simulink model "torqueBalancingJointControl"  (Simulink 8.0)
settings: Solver=FixedStepDiscrete  StartTime=0.0  StopTime=simulationTime  FixedStep=Ts  RelTol=1e-3
InitFcn:
  | initTorqueBalancingJc;
values from neighbouring files (symbols this model uses):
  WBT_modelName = 'matlabTorqueBalancing'    [initTorqueBalancing.m]
undefined symbols (not defined in the file or in its folder): bVectorConstraints, ConstraintsMatrix, DiscIntNeverNeededParam, gain, LEFT_RIGHT_FOOT_IN_CONTACT, reg, ROBOT_DOF, ROBOT_DOF_FOR_SIMULINK, sat, Ts
libraries: WBToolboxLibrary x56, simulink x2
settings Model: Creator=daniele  LastModifiedBy=gnava
settings DebuggingCC: FcnCallInpInsideContextMsg=EnableAllAsWarning  FrameProcessingCompatibilityMsg=error
settings SFSimCC: SimParseCustomCode=off
settings CodeAppCC: CustomSymbolStrType=$N$R$M_T
settings GRTTargetCC: CodeReplacementLibrary=C89/C90 (ANSI)  CombineOutputUpdateFcns=off  GRTInterface=on

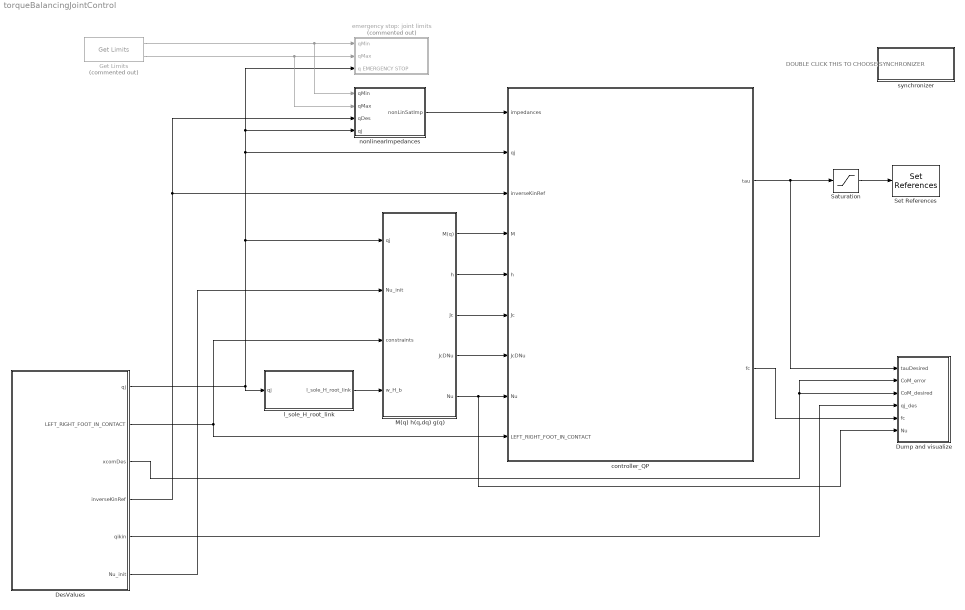
== system torqueBalancingJointControl ==
  note: DOUBLE CLICK THIS TO
      |  CHOOSE SYNCHRONIZER
  DesValues : Subsystem
  Dump and visualize : Subsystem
  Get Limits : WBToolboxLibrary/wholeBodyStates/Get Limits  Commented=on  limitsType=Position  robotName=WBT_robotName  localName=WBT_modelName  wbiFile=WBT_wbiFilename  wbiList=WBT_wbiList
  M(q) h(q,dq) g(q) : Subsystem
  Saturation : Saturate  UpperLimit=sat.torque  LowerLimit=-sat.torque
  Set References : WBToolboxLibrary/wholeBodyActuators/Set References  controlType=Torque  robotName=WBT_robotName  localName=WBT_modelName  wbiFile=WBT_wbiFilename  wbiList=WBT_wbiList
  controller_QP : Subsystem
  emergency stop: joint limits : Subsystem  Commented=on
  l_sole_H_root_link : Subsystem
  nonlinearImpedances : Subsystem
  synchronizer : Subsystem
  wires:
  DesValues/1(qj) -> l_sole_H_root_link/1(qj), M(q) h(q,dq) g(q)/1(qj), controller_QP/2(qj), nonlinearImpedances/4(qj), emergency stop: joint limits/3(q EMERGENCY STOP)
  M(q) h(q,dq) g(q)/1(M(q)) -> controller_QP/4(M)
  Get Limits/1 -> nonlinearImpedances/1(qMin), emergency stop: joint limits/1(qMin)
  M(q) h(q,dq) g(q)/2(h) -> controller_QP/5(h)
  controller_QP/1("tau ") -> Saturation/1, Dump and visualize/1(tauDesired)
  Saturation/1 -> Set References/1
  DesValues/2(LEFT_RIGHT_FOOT_IN_CONTACT) -> controller_QP/9(LEFT_RIGHT_FOOT_IN_CONTACT), M(q) h(q,dq) g(q)/3(constraints)
  nonlinearImpedances/1(nonLinSatImp) -> controller_QP/1(impedances)
  M(q) h(q,dq) g(q)/5(Nu) -> Dump and visualize/6(Nu), controller_QP/8(Nu)
  M(q) h(q,dq) g(q)/3(Jc) -> controller_QP/6(Jc)
  M(q) h(q,dq) g(q)/4(JcDNu) -> controller_QP/7(JcDNu)
  DesValues/4(inverseKinRef) -> controller_QP/3(inverseKinRef), nonlinearImpedances/3(qDes)
  DesValues/5(qikin) -> Dump and visualize/4(qj_des)
  DesValues/3(xcomDes) -> Dump and visualize/2(CoM_error), Dump and visualize/3(CoM_desired)
  controller_QP/2(fc) -> Dump and visualize/5(fc)
  Get Limits/2 -> nonlinearImpedances/2(qMax), emergency stop: joint limits/2(qMax)
  l_sole_H_root_link/1(l_sole_H_root_link) -> M(q) h(q,dq) g(q)/4(w_H_b)
  DesValues/6(Nu_init) -> M(q) h(q,dq) g(q)/2(Nu_init)

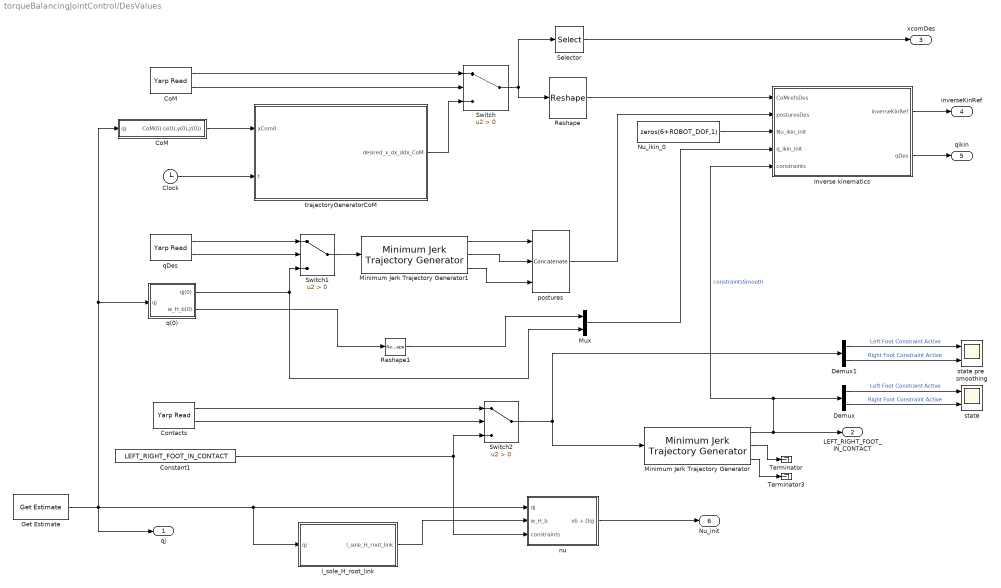
== system torqueBalancingJointControl/DesValues ==
  Clock : Clock
  CoM : WBToolboxLibrary/Utilities/Yarp Read  portName=['/' WBT_modelName '/comDes:i']  signalSize=9  blocking=off  timestamp=off  autoconnect=off  errorOnConnection=on
  "CoM " : Subsystem
  Constant1 : Constant  Value=LEFT_RIGHT_FOOT_IN_CONTACT
  Contacts : WBToolboxLibrary/Utilities/Yarp Read  portName=['/' WBT_modelName '/constraints:i']  signalSize=2  blocking=off  timestamp=off  autoconnect=off  errorOnConnection=on
  Demux : Demux  Outputs=2
  Demux1 : Demux  Outputs=2
  Get Estimate : WBToolboxLibrary/wholeBodyStates/Get Estimate  estimateType=Joints Position  robotName=WBT_robotName  localName=WBT_modelName  wbiFile=WBT_wbiFilename  wbiList=WBT_wbiList
  Inverse kinematics : Subsystem
  Minimum Jerk Trajectory Generator : WBToolboxLibrary/Utilities/Minimum Jerk Trajectory Generator  externalSettlingTime=off  settlingTime=3  sampleTime=Ts  firstDerivatives=on  secondDerivatives=on  explicitInitialValue=off
  Minimum Jerk Trajectory Generator1 : WBToolboxLibrary/Utilities/Minimum Jerk Trajectory Generator  externalSettlingTime=off  settlingTime=3  sampleTime=Ts  firstDerivatives=on  secondDerivatives=on  explicitInitialValue=off
  Mux : Mux  Inputs=2
  Nu_ikin_0 : Constant  Value=zeros(6+ROBOT_DOF,1)
  Reshape : Reshape  OutputDimensionality=Customize  OutputDimensions=[3,3]
  Reshape1 : Reshape
  Selector : Selector  InputPortWidth=9  IndexOptions=Index vector (dialog)  Indices=[1:3]  OutputSizes=1
  Switch : Switch  Criteria=u2 > Threshold
  Switch1 : Switch  Criteria=u2 > Threshold
  Switch2 : Switch  Criteria=u2 > Threshold
  Terminator : Terminator
  Terminator3 : Terminator
  l_sole_H_root_link : Subsystem
  nu : Subsystem
  postures : Concatenate  NumInputs=3  Mode=Multidimensional array  ConcatenateDimension=2
  q(0) : Subsystem
  qDes : WBToolboxLibrary/Utilities/Yarp Read  portName=['/' WBT_modelName '/qDes:i']  signalSize=ROBOT_DOF  blocking=off  timestamp=off  autoconnect=off  errorOnConnection=on
  state : Scope  NumInputPorts=2
      settings: ShowLegends=on  TimeRange=60  YMin=0~0  YMax=2~2
  state pre  smoothing : Scope  NumInputPorts=2
      settings: ShowLegends=on  TimeRange=60  YMin=0~0  YMax=2~2  SaveName=ScopeData7
  trajectoryGeneratorCoM : MATLAB Function  TreatAsAtomicUnit=on
  qj : Outport
  LEFT_RIGHT_FOOT_IN_CONTACT : Outport  Port=2
  xcomDes : Outport  Port=3
  inverseKinRef : Outport  Port=4
  qikin : Outport  Port=5
  Nu_init : Outport  Port=6
  wires:
  Constant1/1 -> Switch2/3, nu/3("constraints ")
  Minimum Jerk Trajectory Generator/1 -> Inverse kinematics/5(constraints), Demux/1, LEFT_RIGHT_FOOT_IN_CONTACT/1  "constraintsSmooth"
  CoM/2 -> Switch/2
  CoM/1 -> Switch/1
  Reshape/1 -> Inverse kinematics/1(CoMrefsDes)
  Switch/1 -> Reshape/1, Selector/1
  qDes/2 -> Switch1/2
  qDes/1 -> Switch1/1
  Selector/1 -> xcomDes/1
  Contacts/2 -> Switch2/2
  Contacts/1 -> Switch2/1
  Switch2/1 -> Demux1/1, Minimum Jerk Trajectory Generator/1
  Demux/1 -> state/1  "Left Foot Constraint Active"
  Demux/2 -> state/2  "Right Foot Constraint Active"
  Demux1/1 -> state pre  smoothing/1  "Left Foot Constraint Active"
  Demux1/2 -> state pre  smoothing/2  "Right Foot Constraint Active"
  "CoM "/1(CoM(0) (x(0),y(0),z(0))) -> trajectoryGeneratorCoM/1(xCom0)
  Clock/1 -> trajectoryGeneratorCoM/2(t)
  trajectoryGeneratorCoM/1(desired_x_dx_ddx_CoM) -> Switch/3
  Switch1/1 -> Minimum Jerk Trajectory Generator1/1
  Minimum Jerk Trajectory Generator1/1 -> postures/1
  Minimum Jerk Trajectory Generator1/2 -> postures/2
  Minimum Jerk Trajectory Generator1/3 -> postures/3
  Nu_ikin_0/1 -> Inverse kinematics/3(Nu_ikin_init)
  Mux/1 -> Inverse kinematics/4(q_ikin_init)
  q(0)/1(qj(0)) -> Mux/2, Switch1/3
  postures/1 -> Inverse kinematics/2(posturesDes)
  Inverse kinematics/2(qDes) -> qikin/1
  Minimum Jerk Trajectory Generator/2 -> Terminator/1
  Minimum Jerk Trajectory Generator/3 -> Terminator3/1
  q(0)/2(w_H_b(0)) -> Reshape1/1
  Reshape1/1 -> Mux/1
  nu/1(vb + Dqj) -> Nu_init/1
  l_sole_H_root_link/1(l_sole_H_root_link) -> nu/2(w_H_b)
  Get Estimate/1 -> qj/1, q(0)/1(qj), "CoM "/1(qj), l_sole_H_root_link/1(qj), nu/1(qj)
  Inverse kinematics/1(inverseKinRef) -> inverseKinRef/1

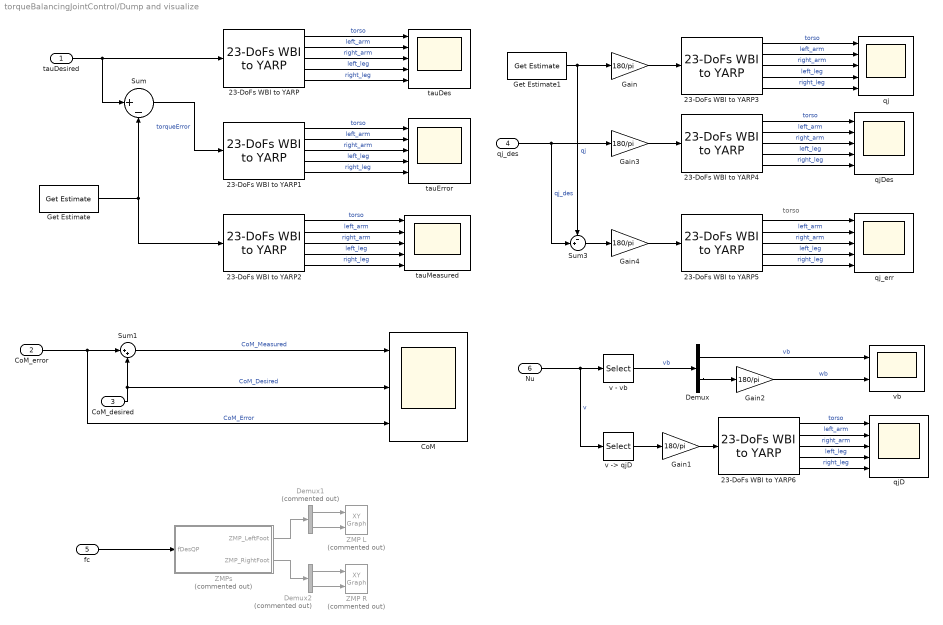
== system torqueBalancingJointControl/Dump and visualize ==
  note: torso
  tauDesired : Inport
  CoM_error : Inport  Port=2
  CoM_desired : Inport  Port=3
  qj_des : Inport  Port=4
  fc : Inport  Port=5
  Nu : Inport  Port=6
  23-DoFs WBI to YARP{,1..6} (7 alike) : WBToolboxLibrary/Utilities/23-DoFs WBI to YARP
  CoM : Scope  NumInputPorts=3
      settings: ShowLegends=on  TimeRange=400  YMin=-0.25~-0.2~-0.2  YMax=1.25~0.6~0.6  SaveName=CoM_data
  Demux : Demux  Outputs=2
  Demux1 : Demux  Commented=on  Outputs=2
  Demux2 : Demux  Commented=on  Outputs=2
  Gain{,1..4} (5 alike) : Gain  Gain=180/pi
  Get Estimate : WBToolboxLibrary/wholeBodyStates/Get Estimate  estimateType=Joints Torque  robotName=WBT_robotName  localName=WBT_modelName  wbiFile=WBT_wbiFilename  wbiList=WBT_wbiList
  Get Estimate1 : WBToolboxLibrary/wholeBodyStates/Get Estimate  estimateType=Joints Position  robotName=WBT_robotName  localName=WBT_modelName  wbiFile=WBT_wbiFilename  wbiList=WBT_wbiList
  Sum : Sum  Inputs=|+-
  Sum1 : Sum  Inputs=|++
  Sum3 : Sum  Inputs=-+|
  ZMP L : simulink/Sinks/XY Graph  Commented=on  xmin=gain.footSize(1,1)  xmax=gain.footSize(1,2)  ymin=gain.footSize(2,1)  ymax=gain.footSize(2,2)  st=-1
  ZMP R : simulink/Sinks/XY Graph  Commented=on  xmin=gain.footSize(1,1)  xmax=gain.footSize(1,2)  ymin=gain.footSize(2,1)  ymax=gain.footSize(2,2)  st=-1
  ZMPs : Subsystem  Commented=on
  qj : Scope  NumInputPorts=5
      settings: ShowLegends=on  TimeRange=40  YMin=-5~-40~-40~-15~-15  YMax=8~60~60~15~15  SaveName=qj_and_v
  qjD : Scope  NumInputPorts=5
      settings: ShowLegends=on  TimeRange=40  YMin=-1~-0.2~-0.6~-3~-3  YMax=3~0.5~0.3~3~3  SaveName=qj_and_v1
  qjDes : Scope  NumInputPorts=5
      settings: ShowLegends=on  TimeRange=40  YMin=-13.18879~-50.35129~-51.01363~-14.07847~-15.42592  YMax=8.56867~62.73253~62.72359~15.05436~15.88206  SaveName=qj_and_v3
  qj_err : Scope  NumInputPorts=5
      settings: ShowLegends=on  TimeRange=40  YMin=-27.27476~-4.23851~-4.57478~-6.37088~-5.38345  YMax=17.10367~4.06727~2.87419~5.35549~6.40509  SaveName=qj_and_v4
  tauDes : Scope  NumInputPorts=5
      settings: ShowLegends=on  TimeRange=14  YMin=-19.49982~-5.04916~-6.41013~-19.61704~-14.11485  YMax=15.70467~4.10511~5.2534~18.2484~18.38621  SaveName=tauDes
  tauError : Scope  NumInputPorts=5
      settings: ShowLegends=on  TimeRange=90  YMin=-4.41555~-1.22651~-0.86191~-3.55477~-4.30808  YMax=5.88399~0.83922~1.20608~5.47683~6.35708  SaveName=tauError
  tauMeasured : Scope  NumInputPorts=5
      settings: ShowLegends=on  TimeRange=14  YMin=-6~-2.5~-2.5~-6~-6  YMax=5~2~1.5~5~5  SaveName=tauMeasured
  v - vb : Selector  InputPortWidth=ROBOT_DOF+6  IndexOptions=Index vector (dialog)  Indices=[1:6]  OutputSizes=1
  "v -> qjD" : Selector  InputPortWidth=ROBOT_DOF+6  IndexOptions=Index vector (dialog)  Indices=[7:ROBOT_DOF+6]  OutputSizes=1
  vb : Scope  NumInputPorts=2
      settings: ShowLegends=on  TimeRange=40  YMin=-0.02~-1.75  YMax=0.0175~2  SaveName=qj_and_v2
  wires:
  CoM_error/1 -> CoM/3, Sum1/1  "CoM_Error"
  CoM_desired/1 -> Sum1/2, CoM/2  "CoM_Desired"
  Sum1/1 -> CoM/1  "CoM_Measured"
  Nu/1 -> "v -> qjD"/1, v - vb/1  "v"
  Get Estimate1/1 -> Sum3/1, Gain/1  "qj"
  Gain/1 -> 23-DoFs WBI to YARP3/1
  23-DoFs WBI to YARP3/5 -> qj/5  "right_leg"
  23-DoFs WBI to YARP3/1 -> qj/1  "torso"
  23-DoFs WBI to YARP3/2 -> qj/2  "left_arm"
  23-DoFs WBI to YARP3/4 -> qj/4  "left_leg"
  23-DoFs WBI to YARP3/3 -> qj/3  "right_arm"
  23-DoFs WBI to YARP6/5 -> qjD/5  "right_leg"
  23-DoFs WBI to YARP6/1 -> qjD/1  "torso"
  23-DoFs WBI to YARP6/2 -> qjD/2  "left_arm"
  23-DoFs WBI to YARP6/4 -> qjD/4  "left_leg"
  23-DoFs WBI to YARP6/3 -> qjD/3  "right_arm"
  "v -> qjD"/1 -> Gain1/1
  v - vb/1 -> Demux/1  "vb"
  Demux/1 -> vb/1  "vb"
  Demux/2 -> Gain2/1
  Gain1/1 -> 23-DoFs WBI to YARP6/1
  Gain2/1 -> vb/2  "wb"
  fc/1 -> ZMPs/1(fDesQP)
  ZMPs/1(ZMP_LeftFoot) -> Demux1/1
  ZMPs/2(ZMP_RightFoot) -> Demux2/1
  Demux1/1 -> ZMP L/1
  Demux1/2 -> ZMP L/2
  Demux2/1 -> ZMP R/1
  Demux2/2 -> ZMP R/2
  tauDesired/1 -> Sum/1, 23-DoFs WBI to YARP/1
  Get Estimate/1 -> 23-DoFs WBI to YARP2/1, Sum/2
  23-DoFs WBI to YARP/5 -> tauDes/5  "right_leg"
  23-DoFs WBI to YARP/1 -> tauDes/1  "torso"
  23-DoFs WBI to YARP/2 -> tauDes/2  "left_arm"
  23-DoFs WBI to YARP/4 -> tauDes/4  "left_leg"
  23-DoFs WBI to YARP/3 -> tauDes/3  "right_arm"
  23-DoFs WBI to YARP1/5 -> tauError/5  "right_leg"
  23-DoFs WBI to YARP1/1 -> tauError/1  "torso"
  23-DoFs WBI to YARP1/2 -> tauError/2  "left_arm"
  23-DoFs WBI to YARP1/4 -> tauError/4  "left_leg"
  23-DoFs WBI to YARP1/3 -> tauError/3  "right_arm"
  Sum/1 -> 23-DoFs WBI to YARP1/1  "torqueError"
  23-DoFs WBI to YARP2/5 -> tauMeasured/5  "right_leg"
  23-DoFs WBI to YARP2/1 -> tauMeasured/1  "torso"
  23-DoFs WBI to YARP2/2 -> tauMeasured/2  "left_arm"
  23-DoFs WBI to YARP2/4 -> tauMeasured/4  "left_leg"
  23-DoFs WBI to YARP2/3 -> tauMeasured/3  "right_arm"
  23-DoFs WBI to YARP4/5 -> qjDes/5  "right_leg"
  23-DoFs WBI to YARP4/1 -> qjDes/1  "torso"
  23-DoFs WBI to YARP4/2 -> qjDes/2  "left_arm"
  23-DoFs WBI to YARP4/4 -> qjDes/4  "left_leg"
  23-DoFs WBI to YARP4/3 -> qjDes/3  "right_arm"
  Gain4/1 -> 23-DoFs WBI to YARP5/1
  23-DoFs WBI to YARP5/5 -> qj_err/5  "right_leg"
  23-DoFs WBI to YARP5/2 -> qj_err/2  "left_arm"
  23-DoFs WBI to YARP5/4 -> qj_err/4  "left_leg"
  23-DoFs WBI to YARP5/3 -> qj_err/3  "right_arm"
  Sum3/1 -> Gain4/1
  qj_des/1 -> Gain3/1, Sum3/2  "qj_des"
  Gain3/1 -> 23-DoFs WBI to YARP4/1
  23-DoFs WBI to YARP5/1 -> qj_err/1

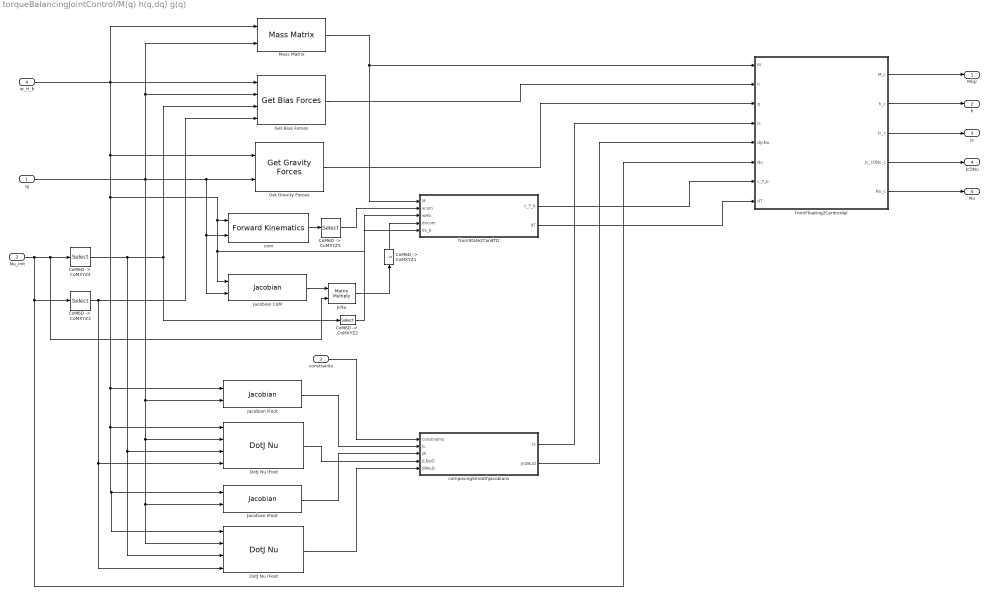
== system torqueBalancingJointControl/M(q) h(q,dq) g(q) ==
  qj : Inport
  Nu_init : Inport  Port=2
  constraints : Inport  Port=3
  w_H_b : Inport  Port=4
  "CoM6D ->  CoMXYZ1" : Selector  InputPortWidth=6  IndexOptions=Index vector (dialog)  Indices=[1 2 3]  OutputSizes=1
  "CoM6D ->  CoMXYZ2" : Selector  InputPortWidth=6  IndexOptions=Index vector (dialog)  Indices=[1 2 3]  OutputSizes=1
  "CoM6D ->  CoMXYZ3" : Selector  InputPortWidth=6+ROBOT_DOF  IndexOptions=Index vector (dialog)  Indices=[7:6+ROBOT_DOF]  OutputSizes=1
  "CoM6D ->  CoMXYZ4" : Selector  InputPortWidth=6+ROBOT_DOF  IndexOptions=Index vector (dialog)  Indices=[1 2 3 4 5 6]  OutputSizes=1
  "CoM6D ->  CoMXYZ5" : Selector  NumberOfDimensions=2  InputPortWidth=7  IndexOptions=Index vector (dialog),Index vector (dialog)  Indices=[1 2 3],[4]  OutputSizes=1,1
  DotJ Nu lFoot : WBToolboxLibrary/wholeBodyModel/Jacobians/DotJ Nu  frameName='l_sole'  robotName=WBT_robotName  localName=WBT_modelName  wbiFile=WBT_wbiFilename  wbiList=WBT_wbiList
  DotJ Nu rFoot : WBToolboxLibrary/wholeBodyModel/Jacobians/DotJ Nu  frameName='r_sole'  robotName=WBT_robotName  localName=WBT_modelName  wbiFile=WBT_wbiFilename  wbiList=WBT_wbiList
  Get Bias Forces : WBToolboxLibrary/wholeBodyModel/Dynamics/Get Bias Forces  robotName=WBT_robotName  localName=WBT_modelName  wbiFile=WBT_wbiFilename  wbiList=WBT_wbiList
  Get Gravity Forces : WBToolboxLibrary/wholeBodyModel/Dynamics/Get Gravity Forces  robotName=WBT_robotName  localName=WBT_modelName  wbiFile=WBT_wbiFilename  wbiList=WBT_wbiList
  Jacobian CoM : WBToolboxLibrary/wholeBodyModel/Jacobians/Jacobian  frameName='com'  robotName=WBT_robotName  localName=WBT_modelName  wbiFile=WBT_wbiFilename  wbiList=WBT_wbiList
  Jacobian lFoot : WBToolboxLibrary/wholeBodyModel/Jacobians/Jacobian  frameName='l_sole'  robotName=WBT_robotName  localName=WBT_modelName  wbiFile=WBT_wbiFilename  wbiList=WBT_wbiList
  Jacobian rFoot : WBToolboxLibrary/wholeBodyModel/Jacobians/Jacobian  frameName='r_sole'  robotName=WBT_robotName  localName=WBT_modelName  wbiFile=WBT_wbiFilename  wbiList=WBT_wbiList
  JcNu : Product  Multiplication=Matrix(*)
  Mass Matrix : WBToolboxLibrary/wholeBodyModel/Dynamics/Mass Matrix  robotName=WBT_robotName  localName=WBT_modelName  wbiFile=WBT_wbiFilename  wbiList=WBT_wbiList
  com : WBToolboxLibrary/wholeBodyModel/Kinematics/Forward Kinematics  frameName='com'  robotName=WBT_robotName  localName=WBT_modelName  wbiFile=WBT_wbiFilename  wbiList=WBT_wbiList
  composingSmoothJacobians : MATLAB Function  TreatAsAtomicUnit=on
  fromFloating2Centroidal : MATLAB Function  TreatAsAtomicUnit=on
  fromState2TandTD : MATLAB Function  TreatAsAtomicUnit=on
  M(q) : Outport
  h : Outport  Port=2
  Jc : Outport  Port=3
  JcDNu : Outport  Port=4
  Nu : Outport  Port=5
  wires:
  w_H_b/1 -> fromState2TandTD/3(wHb), Jacobian CoM/1, com/1, DotJ Nu lFoot/1, Jacobian rFoot/1, DotJ Nu rFoot/1, Jacobian lFoot/1, Get Gravity Forces/1, Get Bias Forces/1, Mass Matrix/1
  qj/1 -> Jacobian lFoot/2, DotJ Nu lFoot/2, Jacobian rFoot/2, DotJ Nu rFoot/2, Get Bias Forces/2, Mass Matrix/2, Jacobian CoM/2, com/2, Get Gravity Forces/2
  "CoM6D ->  CoMXYZ4"/1 -> DotJ Nu rFoot/3, DotJ Nu lFoot/3, "CoM6D ->  CoMXYZ2"/1, Get Bias Forces/3
  "CoM6D ->  CoMXYZ3"/1 -> DotJ Nu rFoot/4, DotJ Nu lFoot/4, Get Bias Forces/4
  Mass Matrix/1 -> fromFloating2Centroidal/1(M), fromState2TandTD/1(M)
  Get Bias Forces/1 -> fromFloating2Centroidal/2(h)
  Get Gravity Forces/1 -> fromFloating2Centroidal/3(g)
  composingSmoothJacobians/1(Jc) -> fromFloating2Centroidal/4(Jc)
  Jacobian lFoot/1 -> composingSmoothJacobians/2(JL)
  Jacobian rFoot/1 -> composingSmoothJacobians/3(JR)
  DotJ Nu lFoot/1 -> composingSmoothJacobians/4(JLNuD)
  DotJ Nu rFoot/1 -> composingSmoothJacobians/5(JRNuD)
  fromFloating2Centroidal/1(M_c) -> M(q)/1
  fromFloating2Centroidal/2(h_c) -> h/1
  fromFloating2Centroidal/3(Jc_c) -> Jc/1
  fromFloating2Centroidal/4(Jc_cDNu_c) -> JcDNu/1
  fromFloating2Centroidal/5(Nu_c) -> Nu/1
  composingSmoothJacobians/2(JcDNuD) -> fromFloating2Centroidal/5(dJcNu)
  com/1 -> "CoM6D ->  CoMXYZ5"/1
  "CoM6D ->  CoMXYZ5"/1 -> fromState2TandTD/2(xcom)
  Jacobian CoM/1 -> JcNu/1
  JcNu/1 -> "CoM6D ->  CoMXYZ1"/1
  "CoM6D ->  CoMXYZ1"/1 -> fromState2TandTD/4(dxcom)
  fromState2TandTD/1(c_T_b) -> fromFloating2Centroidal/7(c_T_b)
  fromState2TandTD/2(dT) -> fromFloating2Centroidal/8(dT)
  "CoM6D ->  CoMXYZ2"/1 -> fromState2TandTD/5(dx_b)
  constraints/1 -> composingSmoothJacobians/1(constraints)
  Nu_init/1 -> fromFloating2Centroidal/6(Nu), "CoM6D ->  CoMXYZ3"/1, JcNu/2, "CoM6D ->  CoMXYZ4"/1

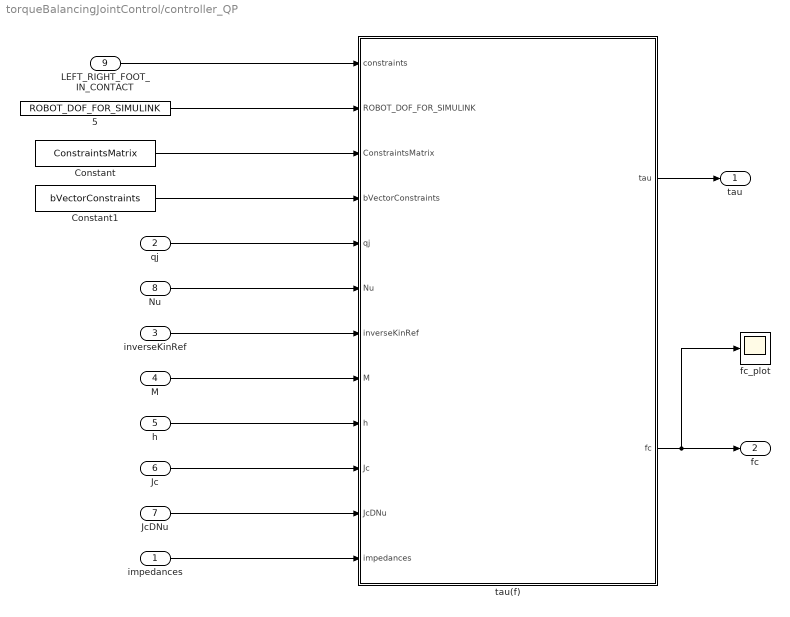
== system torqueBalancingJointControl/controller_QP ==
  impedances : Inport
  qj : Inport  Port=2
  inverseKinRef : Inport  Port=3
  M : Inport  Port=4
  h : Inport  Port=5
  Jc : Inport  Port=6
  JcDNu : Inport  Port=7
  Nu : Inport  Port=8
  LEFT_RIGHT_FOOT_IN_CONTACT : Inport  Port=9
  "    5" : Constant  Value=ROBOT_DOF_FOR_SIMULINK
  Constant : Constant  Value=ConstraintsMatrix
  Constant1 : Constant  Value=bVectorConstraints
  fc_plot : Scope
      settings: YMin=-20  YMax=190  SaveName=ScopeData5
  "tau(f) " : MATLAB Function  TreatAsAtomicUnit=on
  "tau " : Outport
  fc : Outport  Port=2
  wires:
  LEFT_RIGHT_FOOT_IN_CONTACT/1 -> "tau(f) "/1(constraints)
  M/1 -> "tau(f) "/8(M)
  h/1 -> "tau(f) "/9(h)
  "    5"/1 -> "tau(f) "/2(ROBOT_DOF_FOR_SIMULINK)
  Constant/1 -> "tau(f) "/3(ConstraintsMatrix)
  Constant1/1 -> "tau(f) "/4(bVectorConstraints)
  Jc/1 -> "tau(f) "/10(Jc)
  JcDNu/1 -> "tau(f) "/11(JcDNu)
  Nu/1 -> "tau(f) "/6(Nu)
  impedances/1 -> "tau(f) "/12(impedances)
  "tau(f) "/1(tau) -> "tau "/1
  qj/1 -> "tau(f) "/5(qj)
  inverseKinRef/1 -> "tau(f) "/7(inverseKinRef)
  "tau(f) "/2(fc) -> fc_plot/1, fc/1

== system torqueBalancingJointControl/emergency stop: joint limits ==
  qMin : Inport
  qMax : Inport  Port=2
  q EMERGENCY STOP : Inport  Port=3
  Assertion : Assertion  Enabled=on  StopWhenAssertionFail=off
  MATLAB Function : MATLAB Function  TreatAsAtomicUnit=on
  index1 : Constant  Value=0.01  VectorParams1D=off
  wires:
  qMin/1 -> MATLAB Function/1(umin)
  qMax/1 -> MATLAB Function/2(umax)
  index1/1 -> MATLAB Function/4(tol)
  q EMERGENCY STOP/1 -> MATLAB Function/3(u)
  MATLAB Function/1(inRange) -> Assertion/1

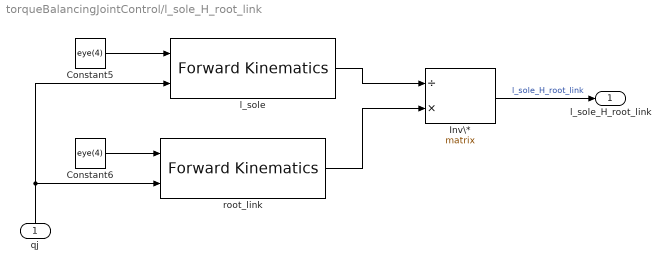
== system torqueBalancingJointControl/l_sole_H_root_link ==
  qj : Inport
  Constant5 : Constant  Value=eye(4)
  Constant6 : Constant  Value=eye(4)
  Inv\* : Product  Inputs=/*  Multiplication=Matrix(*)
  l_sole : WBToolboxLibrary/wholeBodyModel/Kinematics/Forward Kinematics  frameName='l_sole'  robotName=WBT_robotName  localName=WBT_modelName  wbiFile=WBT_wbiFilename  wbiList=WBT_wbiList
  root_link : WBToolboxLibrary/wholeBodyModel/Kinematics/Forward Kinematics  frameName='root_link'  robotName=WBT_robotName  localName=WBT_modelName  wbiFile=WBT_wbiFilename  wbiList=WBT_wbiList
  l_sole_H_root_link : Outport
  wires:
  Constant5/1 -> l_sole/1
  Inv\*/1 -> l_sole_H_root_link/1  "l_sole_H_root_link"
  l_sole/1 -> Inv\*/1
  Constant6/1 -> root_link/1
  qj/1 -> l_sole/2, root_link/2
  root_link/1 -> Inv\*/2

== system torqueBalancingJointControl/nonlinearImpedances ==
  qMin : Inport
  qMax : Inport  Port=2
  qDes : Inport  Port=3
  qj : Inport  Port=4
  nonlinearImpedances : Scope
      settings: ShowLegends=on  TimeRange=25  YMin=-50  YMax=50
  "nonlinearPosturalGains " : MATLAB Function  TreatAsAtomicUnit=on
  nonLinSatImp : Outport
  wires:
  "nonlinearPosturalGains "/1(nonlinearImpedences) -> nonLinSatImp/1, nonlinearImpedances/1
  qMin/1 -> "nonlinearPosturalGains "/3(qMin)
  qMax/1 -> "nonlinearPosturalGains "/4(qMax)
  qj/1 -> "nonlinearPosturalGains "/2(q)
  qDes/1 -> "nonlinearPosturalGains "/1(qDes)

== system torqueBalancingJointControl/synchronizer ==
  Real Time Synchronizer : WBToolboxLibrary/Utilities/Real Time Synchronizer  period=Ts
  Simulator Synchronizer : WBToolboxLibrary/Utilities/Simulator Synchronizer  Commented=on  period=Ts  serverPortName='/clock/rpc'  clientPortName='/WBT_synchronizer/rpc:o'

== system torqueBalancingJointControl/DesValues/CoM  ==
  qj : Inport
  "CoM6D ->  CoMXYZ2" : Selector  NumberOfDimensions=2  InputPortWidth=7  IndexOptions=Index vector (dialog),Index vector (dialog)  Indices=[1 2 3],[4]  OutputSizes=1,1
  Forward Kinematics CoM : WBToolboxLibrary/wholeBodyModel/Kinematics/Forward Kinematics  frameName='com'  robotName=WBT_robotName  localName=WBT_modelName  wbiFile=WBT_wbiFilename  wbiList=WBT_wbiList
  "holder " : WBToolboxLibrary/Utilities/holder 
  holder 1 : WBToolboxLibrary/Utilities/holder 
  l_sole_H_root_link : Subsystem
  CoM(0) (x(0),y(0),z(0)) : Outport
  wires:
  "holder "/1 -> CoM(0) (x(0),y(0),z(0))/1
  qj/1 -> holder 1/1
  holder 1/1 -> Forward Kinematics CoM/2, l_sole_H_root_link/1(qj)
  Forward Kinematics CoM/1 -> "CoM6D ->  CoMXYZ2"/1
  l_sole_H_root_link/1(l_sole_H_root_link) -> Forward Kinematics CoM/1
  "CoM6D ->  CoMXYZ2"/1 -> "holder "/1

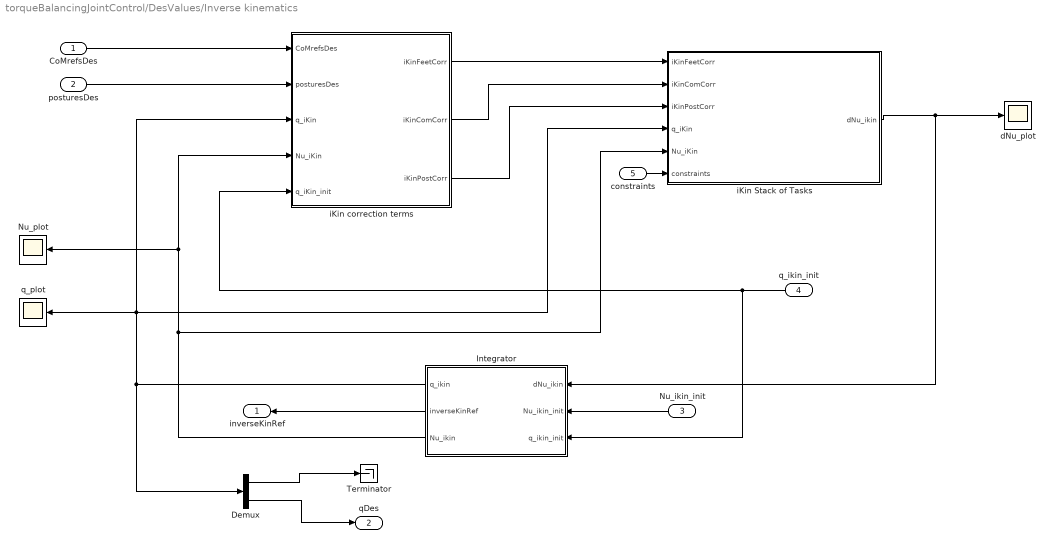
== system torqueBalancingJointControl/DesValues/Inverse kinematics ==
  CoMrefsDes : Inport
  posturesDes : Inport  Port=2
  Nu_ikin_init : Inport  Port=3
  q_ikin_init : Inport  Port=4
  constraints : Inport  Port=5
  Demux : Demux  Outputs=[16;ROBOT_DOF]
  Integrator : Subsystem
  Nu_plot : Scope
      settings: TimeRange=10  YMin=-0.3  YMax=0.3  SaveName=ScopeData3
  Terminator : Terminator
  dNu_plot : Scope
      settings: TimeRange=0.5  YMin=-0.7  YMax=0.7  SaveName=ScopeData2
  iKin Stack of Tasks : Subsystem
  iKin correction terms : Subsystem
  q_plot : Scope
      settings: YMin=-1  YMax=1  SaveName=ScopeData4
  inverseKinRef : Outport
  qDes : Outport  Port=2
  wires:
  CoMrefsDes/1 -> iKin correction terms/1(CoMrefsDes)
  posturesDes/1 -> iKin correction terms/2(posturesDes)
  iKin correction terms/1(iKinFeetCorr) -> iKin Stack of Tasks/1(iKinFeetCorr)
  iKin correction terms/2(iKinComCorr) -> iKin Stack of Tasks/2(iKinComCorr)
  iKin correction terms/3(iKinPostCorr) -> iKin Stack of Tasks/3(iKinPostCorr)
  Integrator/1(q_ikin) -> iKin correction terms/3(q_iKin), iKin Stack of Tasks/4(q_iKin), q_plot/1, Demux/1
  Nu_ikin_init/1 -> Integrator/2(Nu_ikin_init)
  q_ikin_init/1 -> iKin correction terms/5(q_iKin_init), Integrator/3(q_ikin_init)
  Integrator/2(inverseKinRef) -> inverseKinRef/1
  Integrator/3(Nu_ikin) -> Nu_plot/1, iKin correction terms/4(Nu_iKin), iKin Stack of Tasks/5(Nu_iKin)
  iKin Stack of Tasks/1(dNu_ikin) -> Integrator/1(dNu_ikin), dNu_plot/1
  Demux/2 -> qDes/1
  Demux/1 -> Terminator/1
  constraints/1 -> iKin Stack of Tasks/6(constraints)

== system torqueBalancingJointControl/DesValues/l_sole_H_root_link ==
  qj : Inport
  Constant5 : Constant  Value=eye(4)
  Constant6 : Constant  Value=eye(4)
  Inv\* : Product  Inputs=/*  Multiplication=Matrix(*)
  l_sole : WBToolboxLibrary/wholeBodyModel/Kinematics/Forward Kinematics  frameName='l_sole'  robotName=WBT_robotName  localName=WBT_modelName  wbiFile=WBT_wbiFilename  wbiList=WBT_wbiList
  root_link : WBToolboxLibrary/wholeBodyModel/Kinematics/Forward Kinematics  frameName='root_link'  robotName=WBT_robotName  localName=WBT_modelName  wbiFile=WBT_wbiFilename  wbiList=WBT_wbiList
  l_sole_H_root_link : Outport
  wires:
  Constant5/1 -> l_sole/1
  Inv\*/1 -> l_sole_H_root_link/1  "l_sole_H_root_link"
  l_sole/1 -> Inv\*/1
  Constant6/1 -> root_link/1
  qj/1 -> l_sole/2, root_link/2
  root_link/1 -> Inv\*/2

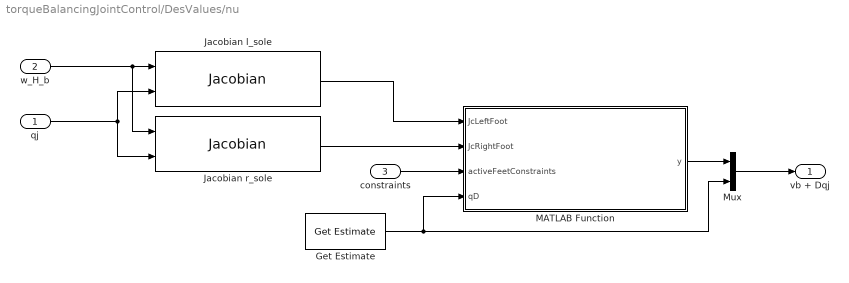
== system torqueBalancingJointControl/DesValues/nu ==
  qj : Inport
  w_H_b : Inport  Port=2
  "constraints " : Inport  Port=3
  Get Estimate : WBToolboxLibrary/wholeBodyStates/Get Estimate  estimateType=Joints Velocity  robotName=WBT_robotName  localName=WBT_modelName  wbiFile=WBT_wbiFilename  wbiList=WBT_wbiList
  Jacobian l_sole : WBToolboxLibrary/wholeBodyModel/Jacobians/Jacobian  frameName='l_sole'  robotName=WBT_robotName  localName=WBT_modelName  wbiFile=WBT_wbiFilename  wbiList=WBT_wbiList
  Jacobian r_sole : WBToolboxLibrary/wholeBodyModel/Jacobians/Jacobian  frameName='r_sole'  robotName=WBT_robotName  localName=WBT_modelName  wbiFile=WBT_wbiFilename  wbiList=WBT_wbiList
  MATLAB Function : MATLAB Function  TreatAsAtomicUnit=on
  Mux : Mux  Inputs=2
  vb + Dqj : Outport
  wires:
  Get Estimate/1 -> MATLAB Function/4(qD), Mux/2
  Mux/1 -> vb + Dqj/1
  Jacobian r_sole/1 -> MATLAB Function/2(JcRightFoot)
  "constraints "/1 -> MATLAB Function/3(activeFeetConstraints)
  MATLAB Function/1(y) -> Mux/1
  Jacobian l_sole/1 -> MATLAB Function/1(JcLeftFoot)
  qj/1 -> Jacobian l_sole/2, Jacobian r_sole/2
  w_H_b/1 -> Jacobian l_sole/1, Jacobian r_sole/1

== system torqueBalancingJointControl/DesValues/q(0) ==
  qj : Inport
  "holder " : WBToolboxLibrary/Utilities/holder 
  l_sole_H_root_link : Subsystem
  qj(0) : Outport
  w_H_b(0) : Outport  Port=2
  wires:
  qj/1 -> "holder "/1
  "holder "/1 -> qj(0)/1, l_sole_H_root_link/1(qj)
  l_sole_H_root_link/1(l_sole_H_root_link) -> w_H_b(0)/1

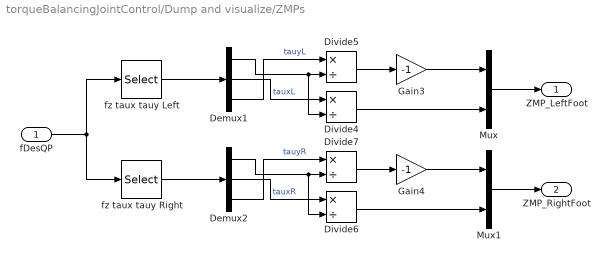
== system torqueBalancingJointControl/Dump and visualize/ZMPs ==
  fDesQP : Inport
  Demux1 : Demux  Outputs=3
  Demux2 : Demux  Outputs=3
  Divide{4..7} (4 alike) : Product  Inputs=*/
  Gain3 : Gain  Gain=-1
  Gain4 : Gain  Gain=-1
  Mux : Mux  Inputs=2
  Mux1 : Mux  Inputs=2
  fz taux tauy Left : Selector  InputPortWidth=12  IndexOptions=Index vector (dialog)  Indices=[3 4 5]  OutputSizes=1
  fz taux tauy Right : Selector  InputPortWidth=12  IndexOptions=Index vector (dialog)  Indices=[9 10 11]  OutputSizes=1
  ZMP_LeftFoot : Outport
  ZMP_RightFoot : Outport  Port=2
  wires:
  fz taux tauy Left/1 -> Demux1/1
  Demux1/1 -> Divide4/2, Divide5/2
  Divide7/1 -> Gain4/1
  Divide4/1 -> Mux/2
  Divide5/1 -> Gain3/1
  fz taux tauy Right/1 -> Demux2/1
  Demux2/1 -> Divide6/2, Divide7/2
  fDesQP/1 -> fz taux tauy Left/1, fz taux tauy Right/1
  Gain3/1 -> Mux/1
  Mux/1 -> ZMP_LeftFoot/1
  Divide6/1 -> Mux1/2
  Gain4/1 -> Mux1/1
  Mux1/1 -> ZMP_RightFoot/1
  Demux1/2 -> Divide4/1  "tauxL"
  Demux1/3 -> Divide5/1  "tauyL"
  Demux2/2 -> Divide6/1  "tauxR"
  Demux2/3 -> Divide7/1  "tauyR"

== system torqueBalancingJointControl/DesValues/CoM /l_sole_H_root_link ==
  qj : Inport
  Constant5 : Constant  Value=eye(4)
  Constant6 : Constant  Value=eye(4)
  Inv\* : Product  Inputs=/*  Multiplication=Matrix(*)
  l_sole : WBToolboxLibrary/wholeBodyModel/Kinematics/Forward Kinematics  frameName='l_sole'  robotName=WBT_robotName  localName=WBT_modelName  wbiFile=WBT_wbiFilename  wbiList=WBT_wbiList
  root_link : WBToolboxLibrary/wholeBodyModel/Kinematics/Forward Kinematics  frameName='root_link'  robotName=WBT_robotName  localName=WBT_modelName  wbiFile=WBT_wbiFilename  wbiList=WBT_wbiList
  l_sole_H_root_link : Outport
  wires:
  Constant5/1 -> l_sole/1
  Inv\*/1 -> l_sole_H_root_link/1  "l_sole_H_root_link"
  l_sole/1 -> Inv\*/1
  Constant6/1 -> root_link/1
  qj/1 -> l_sole/2, root_link/2
  root_link/1 -> Inv\*/2

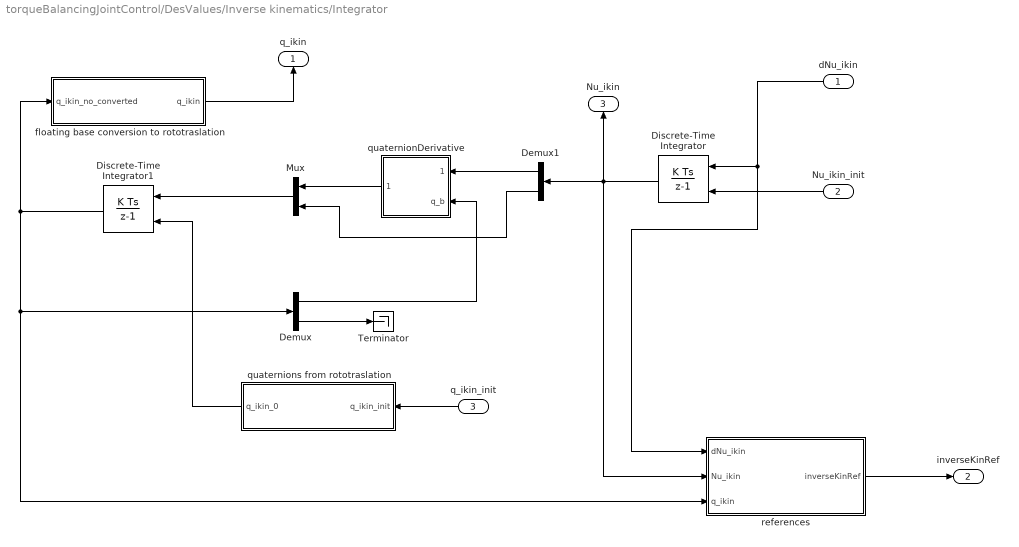
== system torqueBalancingJointControl/DesValues/Inverse kinematics/Integrator ==
  dNu_ikin : Inport
  Nu_ikin_init : Inport  Port=2
  q_ikin_init : Inport  Port=3
  Demux : Demux  Outputs=[7;ROBOT_DOF]
  Demux1 : Demux  Outputs=[6;ROBOT_DOF]
  Discrete-Time Integrator : DiscreteIntegrator  InitialConditionSource=external  SampleTime=Ts  ICPrevOutput=DiscIntNeverNeededParam  ICPrevScaledInput=DiscIntNeverNeededParam
  Discrete-Time Integrator1 : DiscreteIntegrator  InitialConditionSource=external  SampleTime=Ts  ICPrevOutput=DiscIntNeverNeededParam  ICPrevScaledInput=DiscIntNeverNeededParam
  Mux : Mux  Inputs=2
  Terminator : Terminator
  floating base conversion to rototraslation : MATLAB Function  TreatAsAtomicUnit=on
  quaternionDerivative : MATLAB Function  TreatAsAtomicUnit=on
  quaternions from rototraslation : MATLAB Function  TreatAsAtomicUnit=on
  references : MATLAB Function  TreatAsAtomicUnit=on
  q_ikin : Outport
  inverseKinRef : Outport  Port=2
  Nu_ikin : Outport  Port=3
  wires:
  Nu_ikin_init/1 -> Discrete-Time Integrator/2
  q_ikin_init/1 -> quaternions from rototraslation/1(q_ikin_init)
  dNu_ikin/1 -> references/1(dNu_ikin), Discrete-Time Integrator/1
  Demux/2 -> Terminator/1
  Demux/1 -> quaternionDerivative/2(q_b)
  Discrete-Time Integrator1/1 -> references/3(q_ikin), Demux/1, floating base conversion to rototraslation/1(q_ikin_no_converted)
  Discrete-Time Integrator/1 -> references/2(Nu_ikin), Demux1/1, Nu_ikin/1
  Demux1/1 -> quaternionDerivative/1(dNu_b)
  quaternionDerivative/1(dot_qb) -> Mux/1
  Demux1/2 -> Mux/2
  Mux/1 -> Discrete-Time Integrator1/1
  references/1(inverseKinRef) -> inverseKinRef/1
  floating base conversion to rototraslation/1(q_ikin) -> q_ikin/1
  quaternions from rototraslation/1(q_ikin_0) -> Discrete-Time Integrator1/2

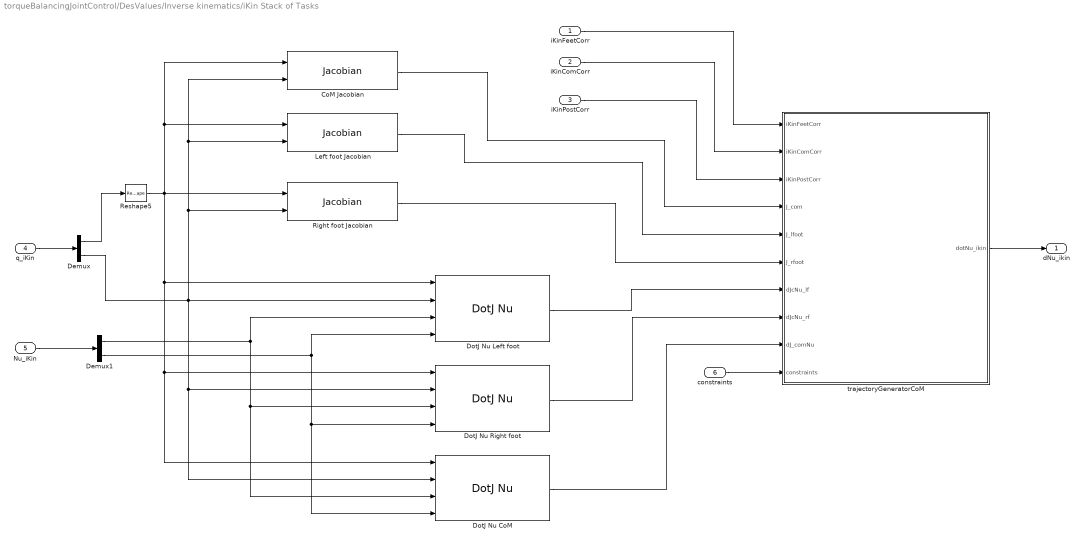
== system torqueBalancingJointControl/DesValues/Inverse kinematics/iKin Stack of Tasks ==
  iKinFeetCorr : Inport
  iKinComCorr : Inport  Port=2
  iKinPostCorr : Inport  Port=3
  q_iKin : Inport  Port=4
  Nu_iKin : Inport  Port=5
  constraints : Inport  Port=6
  CoM Jacobian : WBToolboxLibrary/wholeBodyModel/Jacobians/Jacobian  frameName='com'  robotName=WBT_robotName  localName=WBT_modelName  wbiFile=WBT_wbiFilename  wbiList=WBT_wbiList
  Demux : Demux  Outputs=[16;ROBOT_DOF]
  Demux1 : Demux  Outputs=[6;ROBOT_DOF]
  DotJ Nu CoM : WBToolboxLibrary/wholeBodyModel/Jacobians/DotJ Nu  frameName='com'  robotName=WBT_robotName  localName=WBT_modelName  wbiFile=WBT_wbiFilename  wbiList=WBT_wbiList
  DotJ Nu Left foot : WBToolboxLibrary/wholeBodyModel/Jacobians/DotJ Nu  frameName='l_sole'  robotName=WBT_robotName  localName=WBT_modelName  wbiFile=WBT_wbiFilename  wbiList=WBT_wbiList
  DotJ Nu Right foot : WBToolboxLibrary/wholeBodyModel/Jacobians/DotJ Nu  frameName='r_sole'  robotName=WBT_robotName  localName=WBT_modelName  wbiFile=WBT_wbiFilename  wbiList=WBT_wbiList
  Left foot Jacobian : WBToolboxLibrary/wholeBodyModel/Jacobians/Jacobian  frameName='l_sole'  robotName=WBT_robotName  localName=WBT_modelName  wbiFile=WBT_wbiFilename  wbiList=WBT_wbiList
  Reshape5 : Reshape  OutputDimensionality=Customize  OutputDimensions=[4,4]
  Right foot Jacobian : WBToolboxLibrary/wholeBodyModel/Jacobians/Jacobian  frameName='r_sole'  robotName=WBT_robotName  localName=WBT_modelName  wbiFile=WBT_wbiFilename  wbiList=WBT_wbiList
  trajectoryGeneratorCoM : MATLAB Function  TreatAsAtomicUnit=on
  dNu_ikin : Outport
  wires:
  trajectoryGeneratorCoM/1(dotNu_ikin) -> dNu_ikin/1
  Left foot Jacobian/1 -> trajectoryGeneratorCoM/5(J_lfoot)
  Right foot Jacobian/1 -> trajectoryGeneratorCoM/6(J_rfoot)
  iKinComCorr/1 -> trajectoryGeneratorCoM/2(iKinComCorr)
  iKinFeetCorr/1 -> trajectoryGeneratorCoM/1(iKinFeetCorr)
  iKinPostCorr/1 -> trajectoryGeneratorCoM/3(iKinPostCorr)
  CoM Jacobian/1 -> trajectoryGeneratorCoM/4(J_com)
  DotJ Nu CoM/1 -> trajectoryGeneratorCoM/9(dJ_comNu)
  DotJ Nu Right foot/1 -> trajectoryGeneratorCoM/8(dJcNu_rf)
  DotJ Nu Left foot/1 -> trajectoryGeneratorCoM/7(dJcNu_lf)
  Nu_iKin/1 -> Demux1/1
  q_iKin/1 -> Demux/1
  Demux/2 -> DotJ Nu CoM/2, DotJ Nu Right foot/2, DotJ Nu Left foot/2, Left foot Jacobian/2, CoM Jacobian/2, Right foot Jacobian/2
  Demux1/2 -> DotJ Nu Left foot/4, DotJ Nu CoM/4, DotJ Nu Right foot/4
  Demux1/1 -> DotJ Nu Left foot/3, DotJ Nu CoM/3, DotJ Nu Right foot/3
  Demux/1 -> Reshape5/1
  Reshape5/1 -> DotJ Nu CoM/1, DotJ Nu Right foot/1, DotJ Nu Left foot/1, Left foot Jacobian/1, CoM Jacobian/1, Right foot Jacobian/1
  constraints/1 -> trajectoryGeneratorCoM/10(constraints)

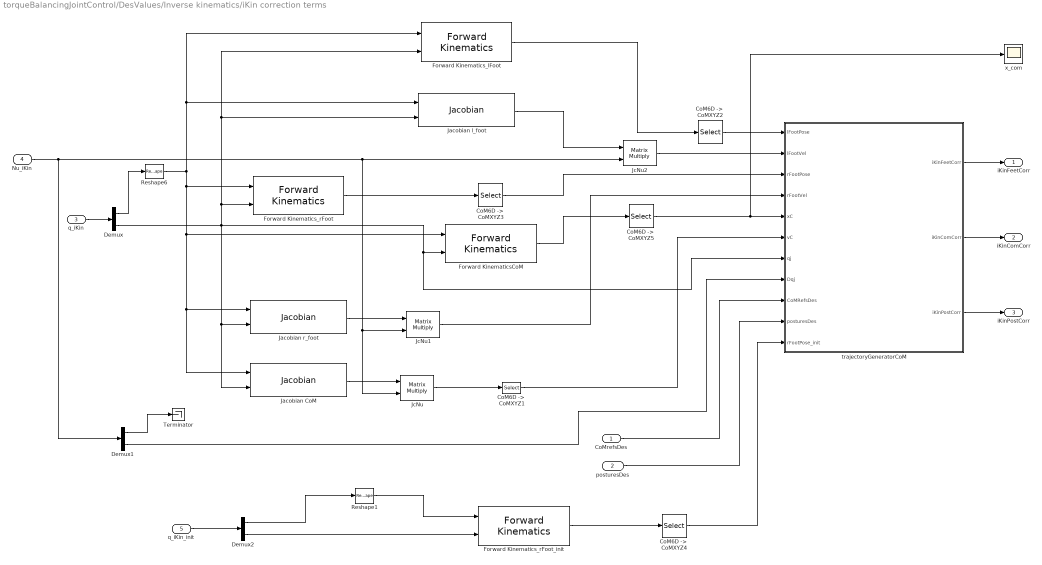
== system torqueBalancingJointControl/DesValues/Inverse kinematics/iKin correction terms ==
  CoMrefsDes : Inport
  posturesDes : Inport  Port=2
  q_iKin : Inport  Port=3
  Nu_iKin : Inport  Port=4
  q_iKin_init : Inport  Port=5
  "CoM6D ->  CoMXYZ1" : Selector  InputPortWidth=6  IndexOptions=Index vector (dialog)  Indices=[1 2 3]  OutputSizes=1
  CoM6D ->  CoMXYZ{2..5} (4 alike) : Selector  NumberOfDimensions=2  InputPortWidth=7  IndexOptions=Index vector (dialog),Index vector (dialog)  Indices=[1 2 3],[4]  OutputSizes=1,1
  Demux : Demux  Outputs=[16;ROBOT_DOF]
  Demux1 : Demux  Outputs=[6,ROBOT_DOF]
  Demux2 : Demux  Outputs=[16;ROBOT_DOF]
  Forward KinematicsCoM : WBToolboxLibrary/wholeBodyModel/Kinematics/Forward Kinematics  frameName='com'  robotName=WBT_robotName  localName=WBT_modelName  wbiFile=WBT_wbiFilename  wbiList=WBT_wbiList
  Forward Kinematics_lFoot : WBToolboxLibrary/wholeBodyModel/Kinematics/Forward Kinematics  frameName='l_sole'  robotName=WBT_robotName  localName=WBT_modelName  wbiFile=WBT_wbiFilename  wbiList=WBT_wbiList
  Forward Kinematics_rFoot : WBToolboxLibrary/wholeBodyModel/Kinematics/Forward Kinematics  frameName='r_sole'  robotName=WBT_robotName  localName=WBT_modelName  wbiFile=WBT_wbiFilename  wbiList=WBT_wbiList
  Forward Kinematics_rFoot_init : WBToolboxLibrary/wholeBodyModel/Kinematics/Forward Kinematics  frameName='r_sole'  robotName=WBT_robotName  localName=WBT_modelName  wbiFile=WBT_wbiFilename  wbiList=WBT_wbiList
  Jacobian CoM : WBToolboxLibrary/wholeBodyModel/Jacobians/Jacobian  frameName='com'  robotName=WBT_robotName  localName=WBT_modelName  wbiFile=WBT_wbiFilename  wbiList=WBT_wbiList
  Jacobian l_foot : WBToolboxLibrary/wholeBodyModel/Jacobians/Jacobian  frameName='l_sole'  robotName=WBT_robotName  localName=WBT_modelName  wbiFile=WBT_wbiFilename  wbiList=WBT_wbiList
  Jacobian r_foot : WBToolboxLibrary/wholeBodyModel/Jacobians/Jacobian  frameName='r_sole'  robotName=WBT_robotName  localName=WBT_modelName  wbiFile=WBT_wbiFilename  wbiList=WBT_wbiList
  JcNu : Product  Multiplication=Matrix(*)
  JcNu1 : Product  Multiplication=Matrix(*)
  JcNu2 : Product  Multiplication=Matrix(*)
  Reshape1 : Reshape  OutputDimensionality=Customize  OutputDimensions=[4,4]
  Reshape6 : Reshape  OutputDimensionality=Customize  OutputDimensions=[4,4]
  Terminator : Terminator
  trajectoryGeneratorCoM : MATLAB Function  TreatAsAtomicUnit=on
  x_com : Scope
      settings: TimeRange=90  YMin=-0.2  YMax=0.6000000000000001  SaveName=ScopeData6
  iKinFeetCorr : Outport
  iKinComCorr : Outport  Port=2
  iKinPostCorr : Outport  Port=3
  wires:
  trajectoryGeneratorCoM/1(iKinFeetCorr) -> iKinFeetCorr/1
  CoMrefsDes/1 -> trajectoryGeneratorCoM/9(CoMRefsDes)
  JcNu/1 -> "CoM6D ->  CoMXYZ1"/1
  posturesDes/1 -> trajectoryGeneratorCoM/10(posturesDes)
  "CoM6D ->  CoMXYZ1"/1 -> trajectoryGeneratorCoM/6(vC)
  JcNu1/1 -> trajectoryGeneratorCoM/4(rFootVel)
  JcNu2/1 -> trajectoryGeneratorCoM/2(lFootVel)
  Nu_iKin/1 -> Demux1/1, JcNu1/2, JcNu/2, JcNu2/2
  q_iKin/1 -> Demux/1
  Jacobian CoM/1 -> JcNu/1
  Forward Kinematics_lFoot/1 -> "CoM6D ->  CoMXYZ2"/1
  Jacobian l_foot/1 -> JcNu2/1
  Jacobian r_foot/1 -> JcNu1/1
  Demux/2 -> Jacobian l_foot/2, Forward Kinematics_lFoot/2, Forward Kinematics_rFoot/2, trajectoryGeneratorCoM/7(qj), Forward KinematicsCoM/2, Jacobian CoM/2, Jacobian r_foot/2
  Demux1/1 -> Terminator/1
  Demux1/2 -> trajectoryGeneratorCoM/8(Dqj)
  q_iKin_init/1 -> Demux2/1
  Demux2/2 -> Forward Kinematics_rFoot_init/2
  Demux2/1 -> Reshape1/1
  Reshape1/1 -> Forward Kinematics_rFoot_init/1
  Demux/1 -> Reshape6/1
  Reshape6/1 -> Jacobian r_foot/1, Jacobian CoM/1, Forward KinematicsCoM/1, Forward Kinematics_rFoot/1, Jacobian l_foot/1, Forward Kinematics_lFoot/1
  "CoM6D ->  CoMXYZ2"/1 -> trajectoryGeneratorCoM/1(lFootPose)
  Forward KinematicsCoM/1 -> "CoM6D ->  CoMXYZ5"/1
  "CoM6D ->  CoMXYZ5"/1 -> x_com/1, trajectoryGeneratorCoM/5(xC)
  Forward Kinematics_rFoot/1 -> "CoM6D ->  CoMXYZ3"/1
  "CoM6D ->  CoMXYZ3"/1 -> trajectoryGeneratorCoM/3(rFootPose)
  Forward Kinematics_rFoot_init/1 -> "CoM6D ->  CoMXYZ4"/1
  "CoM6D ->  CoMXYZ4"/1 -> trajectoryGeneratorCoM/11(rFootPose_init)
  trajectoryGeneratorCoM/2(iKinComCorr) -> iKinComCorr/1
  trajectoryGeneratorCoM/3(iKinPostCorr) -> iKinPostCorr/1

== system torqueBalancingJointControl/DesValues/q(0)/l_sole_H_root_link ==
  qj : Inport
  Constant5 : Constant  Value=eye(4)
  Constant6 : Constant  Value=eye(4)
  Inv\* : Product  Inputs=/*  Multiplication=Matrix(*)
  l_sole : WBToolboxLibrary/wholeBodyModel/Kinematics/Forward Kinematics  frameName='l_sole'  robotName=WBT_robotName  localName=WBT_modelName  wbiFile=WBT_wbiFilename  wbiList=WBT_wbiList
  root_link : WBToolboxLibrary/wholeBodyModel/Kinematics/Forward Kinematics  frameName='root_link'  robotName=WBT_robotName  localName=WBT_modelName  wbiFile=WBT_wbiFilename  wbiList=WBT_wbiList
  l_sole_H_root_link : Outport
  wires:
  Constant5/1 -> l_sole/1
  Inv\*/1 -> l_sole_H_root_link/1  "l_sole_H_root_link"
  l_sole/1 -> Inv\*/1
  Constant6/1 -> root_link/1
  qj/1 -> l_sole/2, root_link/2
  root_link/1 -> Inv\*/2

== matlab function DesValues/Inverse kinematics/Integrator/quaternionDerivative ==
  data: dNu_b input double; dot_qb output double; q_b input double
function dot_qb   = fcn( dNu_b, q_b )

%apply the conversion of reference frame between base and wolrd
omega_b        = dNu_b(4:end);

[~,dcm]        = frame2posrot(q_b);

omega_w        = (dcm')*omega_b;

%calculate the quaternion derivative
quat_base      = q_b(4:end);

dot_qb_b         = quaternionDerivative( omega_w, quat_base );

dot_qb = [dNu_b(1:3);dot_qb_b];

end

== matlab function DesValues/Inverse kinematics/Integrator/floating base conversion to rototraslation ==
  data: q_ikin_no_converted input double; q_ikin output double
function q_ikin = fcn(q_ikin_no_converted)
%#codegen

% define the rototraslation matrix
q_b = q_ikin_no_converted(1:7);

[pos,rot] = frame2posrot(q_b);
Rototr_b  = [rot pos; [0 0 0 1]];

% column-major serialization
vect_R    = Rototr_b(:);

%new state vector
q_ikin    = [vect_R; q_ikin_no_converted(8:end)];

end

== matlab function DesValues/Inverse kinematics/Integrator/quaternions from rototraslation ==
  data: q_ikin_init input double; q_ikin_0 output double
function q_ikin_0 = fcn(q_ikin_init)
%#codegen

q_floating_base = q_ikin_init(1:16);

rot_matrix  = [q_ikin_init(1:3) q_ikin_init(5:7) q_ikin_init(9:11)];

m00 = rot_matrix(1,1);
m11 = rot_matrix(2,2);
m22 = rot_matrix(3,3);

m21 = rot_matrix(3,2);
m12 = rot_matrix(2,3);
m02 = rot_matrix(1,3);
m20 = rot_matrix(3,1);
m10 = rot_matrix(2,1);
m01 = rot_matrix(1,2);

qw = sqrt(1 + m00 + m11 + m22)/2;
qx = (m21 - m12)/( 4 *qw);
qy = (m02 - m20)/( 4 *qw);
qz = (m10 - m01)/( 4 *qw);

quaternions = [qw; qx; qy; qz];

q_ikin_0   =[ q_floating_base(13:15); quaternions; q_ikin_init(17:end)];

end

== matlab function DesValues/Inverse kinematics/Integrator/references ==
  data: dNu_ikin input double; inverseKinRef output double; Nu_ikin input double; q_ikin input double
function inverseKinRef = fcn(dNu_ikin, Nu_ikin, q_ikin)
%#codegen

%composing the joint reference 
ddq_j_ref = dNu_ikin(7:end);
dq_j_ref  = Nu_ikin(7:end);
q_j_ref   = q_ikin(8:end);


inverseKinRef = [q_j_ref dq_j_ref ddq_j_ref];

== matlab function DesValues/Inverse kinematics/iKin Stack of Tasks/trajectoryGeneratorCoM ==
  data: iKinFeetCorr input double; iKinComCorr input double; iKinPostCorr input double; J_com input double; J_lfoot input double; J_rfoot input double; dotNu_ikin output double; dJcNu_lf input double; dJcNu_rf input double; dJ_comNu input double; constraints input double
function dotNu_ikin   = fcn(iKinFeetCorr, iKinComCorr, iKinPostCorr, J_com, J_lfoot, J_rfoot, dJcNu_lf, dJcNu_rf, dJ_comNu, constraints)

%#codegen
n_joints = size(J_com(:,7:end),2);

%% jacobians and their derivatives
Jc   = [constraints(1)*J_lfoot ; constraints(2)*J_rfoot];
Jcom = J_com(1:3,:);
Jp   = [zeros(n_joints,6),eye(n_joints)]; 

dJcNu   = [constraints(1)*dJcNu_lf; constraints(2)*dJcNu_rf];
dJcomNu = dJ_comNu(1:3);

%% state acceleration reference calculation
dotNu_ikin   = Ikin_AccelerationRef_generator(Jc, Jcom, Jp, dJcNu, dJcomNu,iKinFeetCorr, iKinComCorr, iKinPostCorr); 

end

== matlab function DesValues/Inverse kinematics/iKin correction terms/trajectoryGeneratorCoM ==
  data: lFootPose input double; lFootVel input double; rFootPose input double; rFootVel input double; xC input double; vC input double; qj input double; Dqj input double; iKinFeetCorr output double; CoMRefsDes input double; iKinComCorr output double; iKinPostCorr output double; posturesDes input double; gain parameter double; rFootPose_init input double
function [iKinFeetCorr,iKinComCorr,iKinPostCorr]  = fcn(lFootPose,lFootVel,rFootPose,rFootVel,xC,vC,qj,Dqj,CoMRefsDes,posturesDes,gain,rFootPose_init)

%#codegen
delta_rFootPose = rFootPose(1:3)-rFootPose_init;

iKinFeetCorr    = [-gain.ikin.kp*lFootPose(1:3)-gain.ikin.kd*lFootVel(1:3);
                                               -gain.ikin.kd*lFootVel(4:6);
                  -gain.ikin.kp*delta_rFootPose-gain.ikin.kd*rFootVel(1:3);
                                               -gain.ikin.kd*rFootVel(4:6)];
                                         
iKinComCorr  = CoMRefsDes(:,3)-gain.ikin.kp*(xC-CoMRefsDes(:,1))-gain.ikin.kd*(vC-CoMRefsDes(:,2));

iKinPostCorr = posturesDes(:,3)-gain.ikin.kp*(qj-posturesDes(:,1))-gain.ikin.kd*(Dqj-posturesDes(:,2));

end

== matlab function DesValues/nu/MATLAB Function ==
  data: JcLeftFoot input double; JcRightFoot input double; activeFeetConstraints input double; y output double; qD input double; reg parameter double
function y = fcn(JcLeftFoot,JcRightFoot,activeFeetConstraints,qD,reg)
%#codegen

Jc = [activeFeetConstraints(1)*JcLeftFoot;
      activeFeetConstraints(2)*JcRightFoot];

pinvJb = (Jc(:,1:6)'*Jc(:,1:6) + reg.pinvDampVb*eye(6))\Jc(:,1:6)';  
  
% pinvJb = pinv(Jc(:,1:6));

y = -pinvJb*Jc(:,7:end)*qD;

== matlab function DesValues/trajectoryGeneratorCoM ==
  data: desired_x_dx_ddx_CoM output double; xCom0 input double; t input double; references parameter double
function desired_x_dx_ddx_CoM   = fcn(xCom0,t,references)
%#codegen
        
if t > references.noOscillationTime
    A = references.amplitudeOfOscillation;
else
    A = 0;
end
f = references.frequencyOfOscillation;

xcomDes    = xCom0 + A*sin(2*pi*f*t)*references.directionOfOscillation;
% xcomDes(1) =  xcomDes(1) + 0.01;
xDcomDes   =         A*2*pi*f*cos(2*pi*f*t)*references.directionOfOscillation;
xDDcomDes  =        -A*(2*pi*f)^2*sin(2*pi*f*t)*references.directionOfOscillation;

desired_x_dx_ddx_CoM = [xcomDes;xDcomDes;xDDcomDes];

== matlab function M(q) h(q,dq) g(q)/composingSmoothJacobians ==
  data: constraints input double; JL input double; JR input double; Jc output double; JLNuD input double; JRNuD input double; JcDNuD output double
function [Jc, JcDNuD] = composingSmoothJacobians(constraints,JL,JR, JLNuD,JRNuD)
%#codegen
Jc     = [ JL*constraints(1) ;
           JR*constraints(2)];
       
JcDNuD = [ JLNuD*constraints(1) ;
           JRNuD*constraints(2)];

== matlab function M(q) h(q,dq) g(q)/fromFloating2Centroidal ==
  data: M input double; M_c output double; h input double; g input double; Jc input double; dJcNu input double; Nu input double; c_T_b input double; dT input double; h_c output double; Jc_c output double; Jc_cDNu_c output double; Nu_c output double
function [M_c,h_c, Jc_c, Jc_cDNu_c, Nu_c] = fromFloating2Centroidal(M, h, g, Jc, dJcNu, Nu, c_T_b, dT)
%#codegen
[M_c,C_cNu_c, g_c, Jc_c, Jc_cDNu_c, Nu_c] = fromFloatingToCentroidalDynamics(M, h, g, Jc, dJcNu, Nu, c_T_b, dT);
h_c = C_cNu_c + g_c;

== matlab function M(q) h(q,dq) g(q)/fromState2TandTD ==
  data: M input double; xcom input double; c_T_b output double; wHb input double; dxcom input double; dx_b input double; dT output double
function [c_T_b, dT] = centroidalTransformationT_TDot(M,xcom,wHb,dxcom,dx_b)
%#codegen
[c_T_b, dT] = centroidalTransformationT_TDot(xcom,wHb(1:3,4),dxcom,dx_b,M);

== matlab function controller_QP/tau(f)  ==
  data: tau output double; constraints input double; ROBOT_DOF_FOR_SIMULINK input double; ConstraintsMatrix input double; bVectorConstraints input double; qj input double; Nu input double; inverseKinRef input double; M input double; h input double; Jc input double; JcDNu input double; impedances input double; reg parameter double; gain parameter double; fc output double
function [tau,fc]    =  controller(constraints,ROBOT_DOF_FOR_SIMULINK,ConstraintsMatrix,bVectorConstraints,qj,Nu,inverseKinRef, M,h , Jc, JcDNu, impedances,reg,gain)
%#codegen

ROBOT_DOF = size(ROBOT_DOF_FOR_SIMULINK,1);

qTilde    = qj - inverseKinRef(:,1);
qTildeD   = Nu(7:end) - inverseKinRef(:,2);
qDesDD    = inverseKinRef(:,3);
[tau,fc]       = controllerFCN(constraints, ROBOT_DOF, M, h, Jc, JcDNu,impedances, gain.dampings, qTilde,qTildeD, qDesDD,reg);

== matlab function emergency stop: joint limits/MATLAB Function ==
  data: umin input double; umax input double; u input double; inRange output double; tol input double
function inRange = checkRange(umin, umax, u, tol)
%#codegen

res = u < umin + tol | u > umax - tol;
res = sum(res);
if res==0
    inRange = 1;
else
    inRange = 0;
    u < umin + tol | u > umax - tol
end

== matlab function nonlinearImpedances/nonlinearPosturalGains  ==
  data: qDes input double; nonlinearImpedences output double; q input double; qMin input double; qMax input double; gain parameter double
function nonlinearImpedences = fcn(qDes,q,qMin,qMax,gain)
    %#codegen
    qDes = qDes(:,1);
    impedences_at_0     = gain.impedances;
    increasingRatesImp  = (gain.increasingRatesImp)';
    qTildeMax           = gain.qTildeMax;

    tp =  pi./(2*(qMax-qDes));
    tn = -pi./(2*(qMin-qDes));

    
    qTilde = q - qDes;
            
    nonlinearImpedences = (impedences_at_0'   + increasingRatesImp.*tan(pi.*qTilde./(2*qTildeMax)).^2)';
%                                               increasingRatesImp.*tan((tp.*stepFcn(qTilde) + tn.*stepFcn(-qTilde)).*qTilde).^2)';
                                           
end

function y = stepFcn(x) 
   %#codegen
   y = x > 0; 
end
